simulink model "TQ1m1"  (Simulink 8.0)
settings: Solver=ode3  StartTime=0.0  StopTime=inf  FixedStep=0.0025  RelTol=1e-3
undefined symbols (not defined in the file): Serial_Port, sigbuilder_block, Standard_Devices
libraries: rtwinlib x2, simulink x1
Description:
  | Vectorized Quantizer C-MEX S-function
settings Model: Creator=The MathWorks Inc.  LastModifiedBy=x  SimulationMode=external  ExtModeTrigMode=oneshot  ExtModeTrigDuration=10000
settings SolverCC: PositivePriorityOrder=on
settings DataIOCC: LimitDataPoints=off  SignalLoggingSaveFormat=ModelDataLogs
settings OptimizationCC: BlockReduction=off  BooleanDataType=off  InitFltsAndDblsToZero=on
settings DebuggingCC: SaveWithParameterizedLinksMsg=none  SignalResolutionControl=TryResolveAllWithWarning  SolverPrmCheckMsg=none  MultiTaskDSMMsg=warning  MultiTaskCondExecSysMsg=none  FcnCallInpInsideContextMsg=UseLocalSettings
settings HardwareCC: ProdIntDivRoundTo=Zero  ProdEndianess=LittleEndian  ProdHWDeviceType=Generic->32-bit x86 compatible  TargetIntDivRoundTo=Zero  TargetEndianess=LittleEndian  TargetHWDeviceType=MATLAB Host  ProdEqTarget=off
settings SFSimCC: SimCustomHeaderCode=|
  | advapi32.dll
  | comctl32.dll
  | comdlg32.dll
  | gdi32.dll
  | kernel32.dll
  | netapi32.dll
  | shell32.dll
  | shlwapi.dll
  | user32.dll
  | WindowsCodecs.dll
settings SFSimCC: SimUserLibraries=|
  | NtDsAPI.Lib
  | NTMSAPI.Lib
  | NtQuery.Lib
  | windowscodecs.lib
settings RTWCC: SystemTargetFile=rtwin.tlc  TemplateMakefile=rtwin.tmf  Description=Real-Time Windows Target  ProcessScript=rtwin_make_rtw_hook  IncludeERTFirstTime=on  RTWCompilerOptimization=On
settings RTWCC: CustomLibrary=|
  | kernel32.lib
  | kernel32.dll
settings CodeAppCC: MaxIdLength=95
settings RTWinTargetCC: TargetLibSuffix=_rtwin.lib  TargetPreCompLibLocation=C:\Program Files\MATLAB\R2012b\toolbox\rtw\targets\rtwin\lib\win64  CodeReplacementLibrary=ANSI_C  RTWinDir=C:/PROGRA~1/MATLAB/R2012b/toolbox/rtw/targets/rtwin  TargetArch=win64

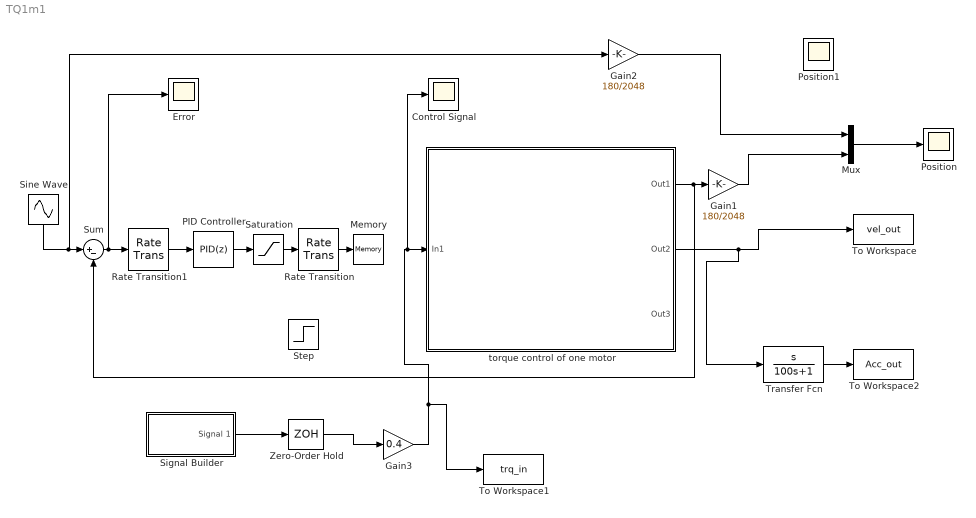
== system TQ1m1 ==
  Control Signal : Scope
      settings: YMin=0.4  YMax=0.4  SaveName=ScopeData7
  Error : Scope
      settings: YMin=2.86  YMax=2.8617  SaveName=ScopeData6
  Gain1 : Gain  Gain=180/2048
  Gain2 : Gain  Gain=180/2048
  Gain3 : Gain  Gain=0.4
  Memory : Memory
  Mux : Mux  Inputs=2
  PID Controller : simulink/Continuous/PID Controller  Controller=PID  TimeDomain=Discrete-time  SampleTime=0.01  IntegratorMethod=Forward Euler  FilterMethod=Forward Euler  Form=Parallel  P=0.002  I=0.01  D=0.00005  N=100  InitialConditionSource=internal  InitialConditionForIntegrator=0  InitialConditionForFilter=0  ExternalReset=none  LimitOutput=off  UpperSaturationLimit=inf  LowerSaturationLimit=-inf  LinearizeAsGain=on  AntiWindupMode=none  Kb=1  TrackingMode=off  Kt=1  PParamMin=[]  PParamMax=[]  IParamMin=[]  IParamMax=[]  DParamMin=[]  DParamMax=[]  NParamMin=[]  NParamMax=[]  KbParamMin=[]  KbParamMax=[]  KtParamMin=[]  KtParamMax=[]  POutMin=[]  POutMax=[]  IOutMin=[]  IOutMax=[]  DOutMin=[]  DOutMax=[]  NOutMin=[]  NOutMax=[]  KbOutMin=[]  KbOutMax=[]  KtOutMin=[]  KtOutMax=[]  IntegratorOutMin=[]  IntegratorOutMax=[]  FilterOutMin=[]  FilterOutMax=[]  SumOutMin=[]  SumOutMax=[]  SumI1OutMin=[]  SumI1OutMax=[]  SumI2OutMin=[]  SumI2OutMax=[]  SumI3OutMin=[]  SumI3OutMax=[]  SumDOutMin=[]  SumDOutMax=[]  SaturationOutMin=[]  SaturationOutMax=[]  IntegratorContinuousStateAttributes=''  IntegratorStateMustResolveToSignalObject=off  IntegratorRTWStateStorageClass=Auto  FilterContinuousStateAttributes=''  FilterStateMustResolveToSignalObject=off  FilterRTWStateStorageClass=Auto
      link override Filter: IntegratorMethod=Integration: Forward Euler  gainval=1.0  ExternalReset=none  InitialConditionSource=internal  InitialCondition=InitialConditionForFilter  InitialConditionMode=State only (most efficient)  SampleTime=-1  OutMin=FilterOutMin  OutMax=FilterOutMax  OutDataTypeStr=FilterOutDataTypeStr  LimitOutput=off  UpperSaturationLimit=inf  LowerSaturationLimit=-inf  ShowSaturationPort=off  ShowStatePort=off
      link override Filter: StateMustResolveToSignalObject=off  RTWStateStorageClass=Auto
  Position : Scope
      settings: TimeRange=10  YMin=0  YMax=210
  Position1 : Scope
      settings: TimeRange=10  YMin=0  YMax=375  SaveName=ScopeData9
  Rate Transition : RateTransition
  Rate Transition1 : RateTransition  OutPortSampleTime=0.01
  Saturation : Saturate  UpperLimit=6  LowerLimit=-6
  Signal Builder : Subsystem  Tag=STV Subsys  LoadFcn=sigbuilder_block('load');  StartFcn=sigbuilder_block('start');  StopFcn=sigbuilder_block('stop');  ClipboardFcn=sigbuilder_block('clipboard');  mask(Sigbuilder block){}
      mask help: Simulink:masks:SigbuilderBlock_MD
      mask init:
      | if ~strcmp(get_param(bdroot(gcbh),'SimulationStatus'),'stopped') tuvar = sigbuilder_block('maskInit'); end
      settings: CopyFcn=sigbuilder_block('copy');  DeleteFcn=sigbuilder_block('delete');  ModelCloseFcn=sigbuilder_block('modelClose');  PreSaveFcn=sigbuilder_block('preSave');  PauseFcn=sigbuilder_block('pause');  ContinueFcn=sigbuilder_block('continue');  NameChangeFcn=sigbuilder_block('namechange');  OpenFcn=sigbuilder_block('open',[403.5 199.5 550.5 395.25 ]);  CloseFcn=sigbuilder_block('close');
      mask Display: plot(0, 0, 100, 100,[2, 2, 32, 32, 2], [68, 8, 8, 68, 68],[32, 2], [38, 38], [32, 19, 2],[53, 60, 44], [32, 17, 17, 2],[16, 16, 31, 31]);txt = getActiveGroup(gcbh);text(2, 100, txt,'verticalAlignment', 'top');
  Sine Wave : Sin  Amplitude=1000  Bias=1500  Frequency=1.5
  Step : Step  Time=0  After=0
  Sum : Sum  Inputs=|+-
  To Workspace : ToWorkspace  VariableName=vel_out  SampleTime=-1
  To Workspace1 : ToWorkspace  VariableName=trq_in  SampleTime=-1
  To Workspace2 : ToWorkspace  VariableName=Acc_out  SampleTime=-1
  Transfer Fcn : TransferFcn  Numerator=[1 0]  Denominator=[100 1]
  Zero-Order Hold : ZeroOrderHold  SampleTime=0.0025
  torque control of one motor : Subsystem  TreatAsAtomicUnit=on  mask(MX64R Real Time Windows Target){p1=1}
      mask prompts: p1 "Dynamixel ID"
      mask help:
      | This Block is desined for torque control of one motor MX64R Dynamixel in real time workshop
      | please be advised with the following issue:
      | Caution1>> change Status Return Level to 1 in EEprom inorder to receive status packet just for read command.
      | Caution2>> It is recommended that Return Delay Time be set as the minimum value within the allowed range of Main Controller.
      | Caution3>> Total sample time of controlling 1 motor is equal to Ts/2. (Ts is the simulink sample time)
      | Copyright @ Aras Lab.
      mask Display:
      | image(imread('mx64.jpg'))
      | port_label('input',1,'Torque')
      | port_label('output',1,'position')
      | port_label('output',2,'velovity')
      | port_label('output',3,'load')
  wires:
  Sum/1 -> Rate Transition1/1, Error/1
  Mux/1 -> Position/1
  Sine Wave/1 -> Gain2/1, Sum/1
  torque control of one motor/1(Out1) -> Sum/2, Gain1/1
  Signal Builder/1(Signal 1) -> Zero-Order Hold/1
  Zero-Order Hold/1 -> Gain3/1
  Gain3/1 -> Control Signal/1, torque control of one motor/1(In1), To Workspace1/1
  Gain2/1 -> Mux/1
  Gain1/1 -> Mux/2
  torque control of one motor/2(Out2) -> Transfer Fcn/1, To Workspace/1
  Transfer Fcn/1 -> To Workspace2/1
  PID Controller/1 -> Saturation/1
  Saturation/1 -> Rate Transition/1
  Rate Transition/1 -> Memory/1
  Rate Transition1/1 -> PID Controller/1

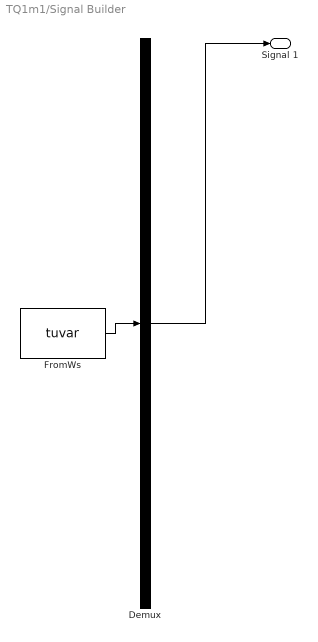
== system TQ1m1/Signal Builder ==
  Demux : Demux  Tag=STV Demux  Outputs=1
  FromWs : FromWorkspace  Tag=STV FromWs  VariableName=tuvar  SampleTime=0  SigBuilderData=DataTag0  VnvData=DataTag1
      SigBuilderData=|
      | common.afterFinalStr = 'Extrapolate'
      | common.sampleTime = 0
      | dataSet.timeRange = [0 20]
      | dataSet.name = 'Group 1'
      | sbobj.Groups.Name = 'Group 1'
      | sbobj.Groups.Signals.Name = 'Signal 1'
      | sbobj.Groups.Signals.XData = [0 0.2 0.2 0.5 0.5 0.6 0.6 0.8 0.8 0.9 0.9 1.4 1.4 1.7 1.7 2 2 2.1 2.1 2.4 2.4 2.7 2.7 2.8 2.8 2.9 2.9 3 3 3.1 3.1 3.2 3.2 3.3 3.3 3.5 3.5 3.7 3.7 3.8 3.8 4 4 4.4 4.4 4.9 4.9 5 5 5.2 5.2 5.3 5.3 5.8 5.8 6.2 6.2 6.3 6.3 6.9 6.9 7 7 7.2 7.2 7.4 7.4 7.8 7.8 7.9 7.9 8 8 8.2 8.2 8.7 8.7 8.8 8.8 9 9 9.1 9.1 9.2 9.2 9.4 9.4 9.5 9.5 9.6 9.6 9.8 9.8 10.1 10.1 10.3 10.3 10.5 10.5 10.7 10.7 10.8 10.8 10.9 10.9 11.2 11.2 11.5 11.5 11.6 11.6 11.7 11.7 11.8 11.8 11.9 11.9 12 12 12.1 12.1 12.5 12.5 12.6 12.6 12.7 12.7 12.9 12.9 13.1 13.1 13.2 13.2 13.8 13.8 14 14 14.1 14.1 14.4 14.4 14.7 14.7 14.9 14.9 15 15 15.2 15.2 15.3 15.3 15.4 15.4 15.7 15.7 15.8 15.8 16.3 16.3 16.5 16.5 16.6 16.6 17 17 17.2 17.2 17.4 17.4 17.5 17.5 17.6 17.6 17.8 17.8 18.1 18.1 18.2 18.2 18.8 18.8 19 19 19.1 19.1 19.2 19.2 19.4 19.4 19.6 19.6 19.7 19.7 19.8 19.8 19.9 19.9 20]
      | sbobj.Groups.Signals.YData = [1 1 -1 -1 1 1 -1 -1 1 1 -1 -1 1 1 -1 -1 1 1 -1 -1 1 1 -1 -1 1 1 -1 -1 1 1 -1 -1 1 1 -1 -1 1 1 -1 -1 1 1 -1 -1 1 1 -1 -1 1 1 -1 -1 1 1 -1 -1 1 1 -1 -1 1 1 -1 -1 1 1 -1 -1 1 1 -1 -1 1 1 -1 -1 1 1 -1 -1 1 1 -1 -1 1 1 -1 -1 1 1 -1 -1 1 1 -1 -1 1 1 -1 -1 1 1 -1 -1 1 1 -1 -1 1 1 -1 -1 1 1 -1 -1 1 1 -1 -1 1 1 -1 -1 1 1 -1 -1 1 1 -1 -1 1 1 -1 -1 1 1 -1 -1 1 1 -1 -1 1 1 -1 -1 1 1 -1 -1 1 1 -1 -1 1 1 -1 -1 1 1 -1 -1 1 1 -1 -1 1 1 -1 -1 1 1 -1 -1 1 1 -1 -1 1 1 -1 -1 1 1 -1 -1 1 1 -1 -1 1 1 -1 -1 1 1]
      | sbobj.Groups.TimeRange = [0 20]
  Signal 1 : Outport  Tag=STV Outport
  wires:
  Demux/1 -> Signal 1/1
  FromWs/1 -> Demux/1

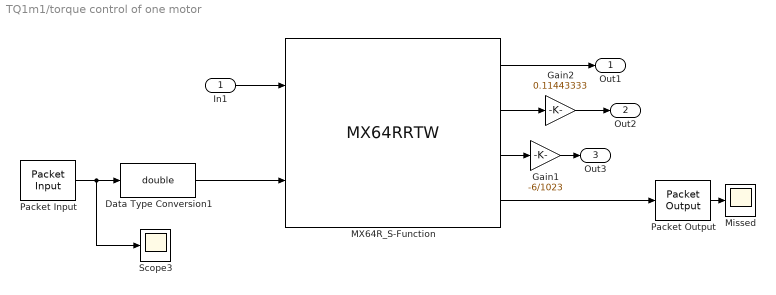
== system TQ1m1/torque control of one motor ==
  In1 : Inport
  Data Type Conversion1 : DataTypeConversion  OutDataTypeStr=double  ConvertRealWorld=Stored Integer (SI)
  Gain1 : Gain  Gain=-6/1023
  Gain2 : Gain  Gain=0.11443333
  MX64R_S-Function : S-Function  FunctionName=MX64RRTW  Parameters=p1  EnableBusSupport=off  mask(S-function: MX64R_RTW){}
      mask Display:
      | port_label('input',1,'desire torque')
      | port_label('input',2,'serial in')
      | port_label('output',1,'position')
      | port_label('output',2,'velocity')
      | port_label('output',3,'load')
      | port_label('output',4,'serial out')
  Missed : Scope
      settings: SaveName=ScopeData8
  Packet Input : rtwinlib/Packet Input  SampleTime=-1  MaxMissedTicks=1000  ShowMissedTicks=off  YieldWhenWaiting=off  DrvName=Standard_Devices/Serial_Port  DrvAddress=10  DrvOptions=[3000000 8 0 0 0 1 0 0]  PacketSize=12  DataTypes='12*uint8'  ShowReady=off  ShowError=off  PacketID=1  ByteOrder=1  ShowTimestamp=off
      settings: AttributesFormatString=Standard Devices\nSerial Port [Ah]
  Packet Output : rtwinlib/Packet Output  SampleTime=-1  MaxMissedTicks=1000  ShowMissedTicks=on  YieldWhenWaiting=off  DrvName=Standard_Devices/Serial_Port  DrvAddress=10  DrvOptions=[3000000 8 0 0 0 1 0 0]  PacketSize=10  DataTypes='10*uint8'  ShowReady=off  ShowError=off  PacketID=1  ByteOrder=1  InitialValue=[]  FinalValue=[]
      settings: AttributesFormatString=Standard Devices\nSerial Port [Ah]
  Scope3 : Scope
      settings: TimeRange=10  YMin=0  YMax=275
  Out1 : Outport  OutMin=[0]  OutMax=[2*pi]
  Out2 : Outport  Port=2
  Out3 : Outport  Port=3
  wires:
  In1/1 -> MX64R_S-Function/1
  Packet Input/1 -> Scope3/1, Data Type Conversion1/1
  Data Type Conversion1/1 -> MX64R_S-Function/2
  MX64R_S-Function/2 -> Gain2/1
  MX64R_S-Function/3 -> Gain1/1
  MX64R_S-Function/4 -> Packet Output/1
  MX64R_S-Function/1 -> Out1/1
  Gain1/1 -> Out3/1
  Gain2/1 -> Out2/1
  Packet Output/1 -> Missed/1
